simulink model "simulacao"  (R2025a)
settings: Solver=VariableStepAuto  StartTime=0.0  StopTime=40  RelTol=1e-3
values from neighbouring files (symbols this model uses):
  b = 0.3    [parametros.m]
  g = 9.81    [parametros.m]
  m = 5    [parametros.m]
settings Model: Creator=luiza  LastModifiedBy=luiza

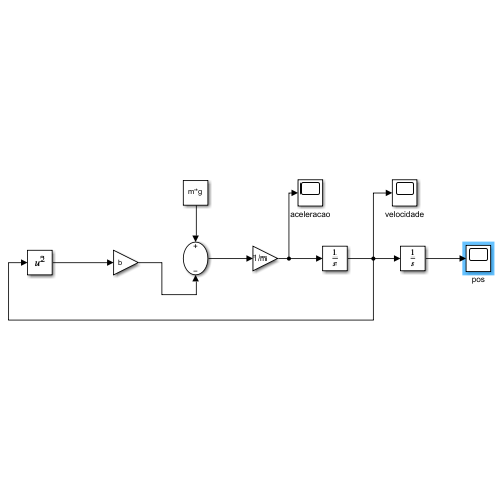
[thumbnail: Simulink's stored preview of the top-level diagram]
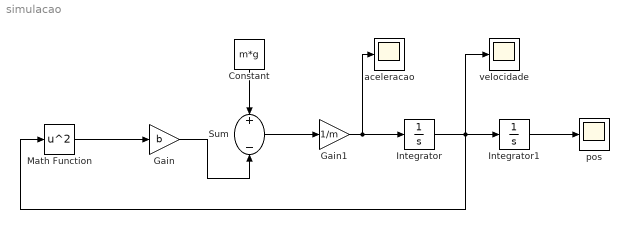
== system simulacao ==
  Constant : Constant  Value=m*g
  Gain : Gain  Gain=b
  Gain1 : Gain  Gain=1/m
  Integrator : Integrator
  Integrator1 : Integrator
  Math Function : Math  Operator=square
  Sum : Sum  Inputs=+-
  aceleracao : Scope
      settings: ActiveDisplayYMinimum=-1.22625  ActiveDisplayYMaximum=11.036250000000003
  pos : Scope
      settings: ActiveDisplayYMinimum=-62.490045613605986  ActiveDisplayYMaximum=562.410410522454
  velocidade : Scope
      settings: ActiveDisplayYMinimum=-1.5983389815680524  ActiveDisplayYMaximum=14.385050834112477  DataLoggingVariableName=ScopeData2
  wires:
  Math Function/1 -> Gain/1
  Constant/1 -> Sum/1
  Gain/1 -> Sum/2
  Sum/1 -> Gain1/1
  Gain1/1 -> aceleracao/1, Integrator/1
  Integrator/1 -> velocidade/1, Integrator1/1, Math Function/1
  Integrator1/1 -> pos/1
